simulink model "controlador_PI"  (R2019a)
settings: Solver=FixedStepAuto  StartTime=0.0  StopTime=20.0  FixedStep=0.01  RelTol=1e-3
libraries: simulink x1
settings Model: Creator=antoniomanuelfr  LastModifiedBy=antoniomanuelfr
settings DataIOCC: ReturnWorkspaceOutputs=off  TimeSaveName=tout_c

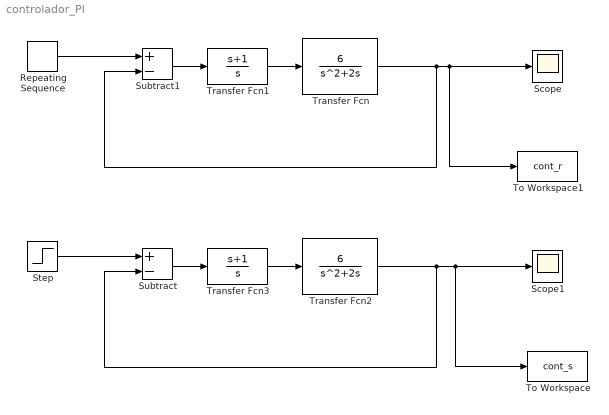
== system controlador_PI ==
  Repeating Sequence : simulink/Sources/Repeating Sequence  rep_seq_t=[0 20]  rep_seq_y=[0 20]
  Scope : Scope
  Scope1 : Scope
  Step : Step  SampleTime=0
  Subtract : Sum  Inputs=+-
  Subtract1 : Sum  Inputs=+-
  To Workspace : ToWorkspace  VariableName=cont_s  SampleTime=-1
  To Workspace1 : ToWorkspace  VariableName=cont_r  SampleTime=-1
  Transfer Fcn : TransferFcn  Numerator=[6]  Denominator=[1 2 0]
  Transfer Fcn1 : TransferFcn  Numerator=[1 1]  Denominator=[1 0]
  Transfer Fcn2 : TransferFcn  Numerator=[6]  Denominator=[1 2 0]
  Transfer Fcn3 : TransferFcn  Numerator=[1 1]  Denominator=[1 0]
  wires:
  Subtract1/1 -> Transfer Fcn1/1
  Transfer Fcn/1 -> Subtract1/2, To Workspace1/1, Scope/1
  Repeating Sequence/1 -> Subtract1/1
  Transfer Fcn1/1 -> Transfer Fcn/1
  Transfer Fcn2/1 -> Subtract/2, To Workspace/1, Scope1/1
  Subtract/1 -> Transfer Fcn3/1
  Step/1 -> Subtract/1
  Transfer Fcn3/1 -> Transfer Fcn2/1
